simulink model "gm_DUALportRAMinterface_v3_vnl"  (R2024a)
settings: Solver=FixedStepDiscrete  StartTime=0.0  StopTime=20  RelTol=1e-3
undefined symbols (not defined in the file or in its folder): magnitude, Ts
libraries: hdlsllib x419, hdlmdlgenlib x103, embmathops x12, simulink x5, dsphdlxfrm2 x2
(part 2 of 11)

== system gm_DUALportRAMinterface_v3_vnl/PL/to_uint32_5 ==
  u_port : Inport  OutDataTypeStr=fixdt(1, 33, 15)  PortDimensions=1  SampleTime=3.00000003e-08
  Bit Concat : hdlsllib/Logic and Bit Operations/Bit Concat  numInputs=18
  Bit Shift1 : hdlsllib/Logic and Bit Operations/Bit Shift  mode=Shift Left Logical  N=15
  Bit Shift19 : hdlsllib/Logic and Bit Operations/Bit Shift  mode=Shift Left Logical  N=1
  Bit Shift2 : hdlsllib/Logic and Bit Operations/Bit Shift  mode=Shift Right Logical  N=16
  Bit Shift20 : hdlsllib/Logic and Bit Operations/Bit Shift  mode=Shift Left Logical  N=10
  Bit Shift21 : hdlsllib/Logic and Bit Operations/Bit Shift  mode=Shift Right Logical  N=1
  Bit Shift22 : hdlsllib/Logic and Bit Operations/Bit Shift  mode=Shift Left Logical  N=11
  Bit Shift23 : hdlsllib/Logic and Bit Operations/Bit Shift  mode=Shift Left Logical  N=12
  Bit Shift24 : hdlsllib/Logic and Bit Operations/Bit Shift  mode=Shift Left Logical  N=13
  Bit Shift25 : hdlsllib/Logic and Bit Operations/Bit Shift  mode=Shift Left Logical  N=14
  Bit Shift26 : hdlsllib/Logic and Bit Operations/Bit Shift  mode=Shift Left Logical  N=2
  Bit Shift27 : hdlsllib/Logic and Bit Operations/Bit Shift  mode=Shift Left Logical  N=3
  Bit Shift28 : hdlsllib/Logic and Bit Operations/Bit Shift  mode=Shift Left Logical  N=4
  Bit Shift29 : hdlsllib/Logic and Bit Operations/Bit Shift  mode=Shift Left Logical  N=5
  Bit Shift30 : hdlsllib/Logic and Bit Operations/Bit Shift  mode=Shift Left Logical  N=6
  Bit Shift31 : hdlsllib/Logic and Bit Operations/Bit Shift  mode=Shift Left Logical  N=7
  Bit Shift32 : hdlsllib/Logic and Bit Operations/Bit Shift  mode=Shift Left Logical  N=8
  Bit Shift33 : hdlsllib/Logic and Bit Operations/Bit Shift  mode=Shift Left Logical  N=9
  Data Type Conversion{1..2,12..16,26,34..43} (18 alike) : DataTypeConversion  OutDataTypeStr=fixdt(0,1,0)  SaturateOnIntegerOverflow=off  RndMeth=Floor
  Data Type Conversion44 : DataTypeConversion  OutDataTypeStr=uint32  SaturateOnIntegerOverflow=off  RndMeth=Floor
  Out1 : Outport  SampleTime=3.00000003e-08
  wires:
  Data Type Conversion44/1 -> Out1/1
  Data Type Conversion43/1 -> Bit Concat/10
  Data Type Conversion42/1 -> Bit Concat/12
  Data Type Conversion41/1 -> Bit Concat/13
  Data Type Conversion40/1 -> Bit Concat/14
  Data Type Conversion39/1 -> Bit Concat/15
  Data Type Conversion38/1 -> Bit Concat/16
  Data Type Conversion37/1 -> Bit Concat/17
  Data Type Conversion36/1 -> Bit Concat/4
  Data Type Conversion35/1 -> Bit Concat/5
  Data Type Conversion34/1 -> Bit Concat/6
  Data Type Conversion26/1 -> Bit Concat/7
  Data Type Conversion2/1 -> Bit Concat/1
  Data Type Conversion16/1 -> Bit Concat/8
  Data Type Conversion15/1 -> Bit Concat/9
  Data Type Conversion14/1 -> Bit Concat/11
  Data Type Conversion13/1 -> Bit Concat/2
  Data Type Conversion12/1 -> Bit Concat/3
  Data Type Conversion1/1 -> Bit Concat/18
  Bit Shift33/1 -> Data Type Conversion42/1
  Bit Shift32/1 -> Data Type Conversion14/1
  Bit Shift31/1 -> Data Type Conversion43/1
  Bit Shift30/1 -> Data Type Conversion15/1
  Bit Shift29/1 -> Data Type Conversion16/1
  Bit Shift28/1 -> Data Type Conversion26/1
  Bit Shift27/1 -> Data Type Conversion34/1
  Bit Shift26/1 -> Data Type Conversion35/1
  Bit Shift25/1 -> Data Type Conversion37/1
  Bit Shift24/1 -> Data Type Conversion38/1
  Bit Shift23/1 -> Data Type Conversion39/1
  Bit Shift22/1 -> Data Type Conversion40/1
  Bit Shift21/1 -> Data Type Conversion13/1
  Bit Shift20/1 -> Data Type Conversion41/1
  Bit Shift2/1 -> Data Type Conversion2/1
  Bit Shift19/1 -> Data Type Conversion36/1
  Bit Shift1/1 -> Data Type Conversion1/1
  Bit Concat/1 -> Data Type Conversion44/1
  u_port/1 -> Bit Shift1/1, Bit Shift19/1, Bit Shift2/1, Bit Shift20/1, Bit Shift21/1, Bit Shift22/1, Bit Shift23/1, Bit Shift24/1, Bit Shift25/1, Bit Shift26/1, Bit Shift27/1, Bit Shift28/1, Bit Shift29/1, Bit Shift30/1, Bit Shift31/1, Bit Shift32/1, Bit Shift33/1, Data Type Conversion12/1

== system gm_DUALportRAMinterface_v3_vnl/PL/to_uint32_6 ==
  u_port : Inport  OutDataTypeStr=fixdt(1, 33, 15)  PortDimensions=1  SampleTime=3.00000003e-08
  Bit Concat : hdlsllib/Logic and Bit Operations/Bit Concat  numInputs=18
  Bit Shift1 : hdlsllib/Logic and Bit Operations/Bit Shift  mode=Shift Left Logical  N=15
  Bit Shift19 : hdlsllib/Logic and Bit Operations/Bit Shift  mode=Shift Left Logical  N=1
  Bit Shift2 : hdlsllib/Logic and Bit Operations/Bit Shift  mode=Shift Right Logical  N=16
  Bit Shift20 : hdlsllib/Logic and Bit Operations/Bit Shift  mode=Shift Left Logical  N=10
  Bit Shift21 : hdlsllib/Logic and Bit Operations/Bit Shift  mode=Shift Right Logical  N=1
  Bit Shift22 : hdlsllib/Logic and Bit Operations/Bit Shift  mode=Shift Left Logical  N=11
  Bit Shift23 : hdlsllib/Logic and Bit Operations/Bit Shift  mode=Shift Left Logical  N=12
  Bit Shift24 : hdlsllib/Logic and Bit Operations/Bit Shift  mode=Shift Left Logical  N=13
  Bit Shift25 : hdlsllib/Logic and Bit Operations/Bit Shift  mode=Shift Left Logical  N=14
  Bit Shift26 : hdlsllib/Logic and Bit Operations/Bit Shift  mode=Shift Left Logical  N=2
  Bit Shift27 : hdlsllib/Logic and Bit Operations/Bit Shift  mode=Shift Left Logical  N=3
  Bit Shift28 : hdlsllib/Logic and Bit Operations/Bit Shift  mode=Shift Left Logical  N=4
  Bit Shift29 : hdlsllib/Logic and Bit Operations/Bit Shift  mode=Shift Left Logical  N=5
  Bit Shift30 : hdlsllib/Logic and Bit Operations/Bit Shift  mode=Shift Left Logical  N=6
  Bit Shift31 : hdlsllib/Logic and Bit Operations/Bit Shift  mode=Shift Left Logical  N=7
  Bit Shift32 : hdlsllib/Logic and Bit Operations/Bit Shift  mode=Shift Left Logical  N=8
  Bit Shift33 : hdlsllib/Logic and Bit Operations/Bit Shift  mode=Shift Left Logical  N=9
  Data Type Conversion{1..2,12..16,26,34..43} (18 alike) : DataTypeConversion  OutDataTypeStr=fixdt(0,1,0)  SaturateOnIntegerOverflow=off  RndMeth=Floor
  Data Type Conversion44 : DataTypeConversion  OutDataTypeStr=uint32  SaturateOnIntegerOverflow=off  RndMeth=Floor
  Out1 : Outport  SampleTime=3.00000003e-08
  wires:
  Data Type Conversion44/1 -> Out1/1
  Data Type Conversion43/1 -> Bit Concat/10
  Data Type Conversion42/1 -> Bit Concat/12
  Data Type Conversion41/1 -> Bit Concat/13
  Data Type Conversion40/1 -> Bit Concat/14
  Data Type Conversion39/1 -> Bit Concat/15
  Data Type Conversion38/1 -> Bit Concat/16
  Data Type Conversion37/1 -> Bit Concat/17
  Data Type Conversion36/1 -> Bit Concat/4
  Data Type Conversion35/1 -> Bit Concat/5
  Data Type Conversion34/1 -> Bit Concat/6
  Data Type Conversion26/1 -> Bit Concat/7
  Data Type Conversion2/1 -> Bit Concat/1
  Data Type Conversion16/1 -> Bit Concat/8
  Data Type Conversion15/1 -> Bit Concat/9
  Data Type Conversion14/1 -> Bit Concat/11
  Data Type Conversion13/1 -> Bit Concat/2
  Data Type Conversion12/1 -> Bit Concat/3
  Data Type Conversion1/1 -> Bit Concat/18
  Bit Shift33/1 -> Data Type Conversion42/1
  Bit Shift32/1 -> Data Type Conversion14/1
  Bit Shift31/1 -> Data Type Conversion43/1
  Bit Shift30/1 -> Data Type Conversion15/1
  Bit Shift29/1 -> Data Type Conversion16/1
  Bit Shift28/1 -> Data Type Conversion26/1
  Bit Shift27/1 -> Data Type Conversion34/1
  Bit Shift26/1 -> Data Type Conversion35/1
  Bit Shift25/1 -> Data Type Conversion37/1
  Bit Shift24/1 -> Data Type Conversion38/1
  Bit Shift23/1 -> Data Type Conversion39/1
  Bit Shift22/1 -> Data Type Conversion40/1
  Bit Shift21/1 -> Data Type Conversion13/1
  Bit Shift20/1 -> Data Type Conversion41/1
  Bit Shift2/1 -> Data Type Conversion2/1
  Bit Shift19/1 -> Data Type Conversion36/1
  Bit Shift1/1 -> Data Type Conversion1/1
  Bit Concat/1 -> Data Type Conversion44/1
  u_port/1 -> Bit Shift1/1, Bit Shift19/1, Bit Shift2/1, Bit Shift20/1, Bit Shift21/1, Bit Shift22/1, Bit Shift23/1, Bit Shift24/1, Bit Shift25/1, Bit Shift26/1, Bit Shift27/1, Bit Shift28/1, Bit Shift29/1, Bit Shift30/1, Bit Shift31/1, Bit Shift32/1, Bit Shift33/1, Data Type Conversion12/1

== system gm_DUALportRAMinterface_v3_vnl/PL_vnl/index_counter ==
  In1 : Inport
  In2 : Inport  Port=2
  Add : Sum  OutDataTypeStr=Inherit: Same as first input
  Constant18 : Constant  OutDataTypeStr=fixdt(0,16,0)  SampleTime=Ts
  Constant19 : Constant  Value=0  OutDataTypeStr=fixdt(0,16,0)  SampleTime=Ts
  Constant20 : Constant  Value=0  OutDataTypeStr=uint16  SampleTime=Ts
  Delay : Delay  DelayLength=1  InitialCondition=0  SampleTime=Ts
  Switch : Switch  Criteria=u2 > Threshold  SaturateOnIntegerOverflow=off  InputSameDT=off  OutDataTypeStr=Inherit: Same as first input
  Switch8 : Switch  Criteria=u2 > Threshold  SaturateOnIntegerOverflow=off  InputSameDT=off  OutDataTypeStr=Inherit: Same as first input
  index_counter : Outport
  wires:
  In1/1 -> Switch/2
  Constant18/1 -> Switch/1
  Constant20/1 -> Switch8/1
  Add/1 -> Delay/1
  In2/1 -> Switch8/2
  Delay/1 -> Switch8/3, index_counter/1
  Switch/1 -> Add/1
  Switch8/1 -> Add/2
  Constant19/1 -> Switch/3

== system gm_DUALportRAMinterface_v3_vnl/PL_vnl/integration_block1 ==
  data_in : Inport
  data_in1 : Inport  Port=2
  start_ga : Inport  Port=3
  D2 : Subsystem
      settings: PortSchema="{\"entries\":[{\"content\":{\"sides\":[{\"content\":{\"connectorIds\":[\"In1\",\"In2\"]},\"type\":\"ConnectorPlacement.EquallySpacedRectSide\",\"uuid\":\"5abe48ab-1b34-4cb0-8d41-07cb17904e64\"},{\"content\":{\"connectorIds\":[\"Out1\"],\"side\":\"RIGHT\"},\"type\":\"ConnectorPlacement.EquallySpacedRectSide\",\"uuid\":\"19bc24ff-88f3-42df-af8e-ecb9c1c6119c\"},{\"content\":{\"connectorIds\":[\"In3\"],\"side\":\"TOP\"},\"type\":\"ConnectorPlacement.EquallySpacedRectSide\",\"uuid\":\"46fc65c4-6cee-4e0a-9107-9d106d0a52a5\"},{\"content\":{\"connectorIds\":[\"In4\"],\"side\":\"BOTTOM\"},\"type\":\"ConnectorPlacement.EquallySpacedRectSide\",\"uuid\":\"10a5fc09-3948-4556-8b0c-050853396926\"}]},\"type\":\"ConnectorPlacement.EquallySpacedConnector\",\"uuid\":\"9cc35bfe-5b00-42b0-9811-425d4f0f8f7b\"}],\"packageUris\":[\"http://schema.mathworks.com/mf0/Connector/R2020b\"],\"version\":\"1.0\"}"
  Delay : Delay  DelayLength=6145  InitialCondition=0  UseCircularBuffer=on  SampleTime=Ts
  Delay3 : Delay  DelayLength=1  InitialCondition=0  SampleTime=Ts
  FFT : dsphdlxfrm2/FFT  Architecture=Burst Radix 2  FFTLengthSource=Property  FFTLength=4096  FFTLengthMax=1024  ComplexMultiplication=Use 4 multipliers and 2 adders  BitReversedOutput=off  BitReversedInput=off  Normalize=off  SimulateUsing=Code generation  RoundingMethod=Floor  ResetInputPort=on  StartOutputPort=off  EndOutputPort=off
  FIFO_system1 : Subsystem
  FIFO_system3 : Subsystem
  GA_main : Subsystem
      settings: PortSchema="{\"entries\":[{\"content\":{\"sides\":[{\"content\":{\"connectorIds\":[\"In1\",\"In2\",\"In3\",\"In4\",\"In5\",\"In6\",\"In7\",\"In8\",\"In9\",\"In10\",\"In11\"]},\"type\":\"ConnectorPlacement.EquallySpacedRectSide\",\"uuid\":\"daccc056-a93f-45e5-9369-71b73e32651e\"},{\"content\":{\"connectorIds\":[\"Out1\",\"Out2\"],\"side\":\"RIGHT\"},\"type\":\"ConnectorPlacement.EquallySpacedRectSide\",\"uuid\":\"82109161-9ebe-455f-914b-56f9927b10eb\"},{\"content\":{\"connectorIds\":[\"Out3\",\"Out4\",\"Out5\",\"In12\",\"In13\"],\"side\":\"TOP\"},\"type\":\"ConnectorPlacement.EquallySpacedRectSide\",\"uuid\":\"07b2e20b-bb92-4769-b746-3d44a115cdd8\"}]},\"type\":\"ConnectorPlacement.EquallySpacedConnector\",\"uuid\":\"c9f522d4-4f80-4900-b8a5-3110692e6ae8\"}],\"packageUris\":[\"http://schema.mathworks.com/mf0/Connector/R2020b\"],\"version\":\"1.0\"}"
  Scope1 : Scope
  Subsystem : Subsystem
  Sum : Sum  Inputs=|+-  OutDataTypeStr=Inherit: Same as first input
  Terminator : Terminator
  Terminator1 : Terminator
  Terminator2 : Terminator
  accumulator_scorer : Subsystem
  ga_done : Outport
  elite_individual : Outport  Port=2
  wires:
  GA_main/1(elite_individual) -> elite_individual/1
  FIFO_system1/4(FIFO_full) -> FIFO_system3/3(load_fifo)
  Subsystem/9(random_sample_out) -> GA_main/11(tb_random_sample)
  Subsystem/8(a4_random_out) -> GA_main/10(a4rnd)
  Subsystem/7(a3_random_out) -> GA_main/9(a3rnd)
  Subsystem/6(a2_random_out) -> GA_main/8(a2rnd)
  Subsystem/5(b4_random_out) -> GA_main/7(b4rnd)
  Subsystem/4(b3_random_out) -> GA_main/6(b3rnd)
  Subsystem/3(b2_random_out) -> GA_main/5(b2rnd)
  Subsystem/2(random_method_out) -> GA_main/4(random_method)
  Subsystem/1(random_gene_out) -> GA_main/3(random_gene)
  Delay/1 -> D2/3(reset_D2)
  Sum/1 -> FFT/1
  FIFO_system3/4(FIFO_full) -> GA_main/12(FIFO_full)
  FIFO_system1/3(reset_fft) -> FFT/3, Delay/1
  FIFO_system1/2(data_valid) -> FFT/2
  data_in1/1 -> FIFO_system3/1(data_in)
  Delay3/1 -> GA_main/13(score_done)
  FIFO_system3/3(reset_fft) -> Terminator2/1
  accumulator_scorer/2(individual_score_valid) -> Delay3/1
  GA_main/3(individual_to_d2) -> D2/4(Individual_input)
  FIFO_system3/1(data_out) -> D2/1(GAerror)
  GA_main/2(ga_done) -> ga_done/1
  data_in/1 -> FIFO_system1/1(data_in)
  GA_main/4(FIFO_out_en) -> FIFO_system1/2(enable_output), FIFO_system3/2(enable_output), D2/2(push_individual)
  GA_main/5(load_fifo) -> FIFO_system1/3(load_fifo)
  FFT/3 -> Terminator/1
  FFT/1 -> accumulator_scorer/1(data_in)
  D2/1(response) -> Sum/2
  start_ga/1 -> Subsystem/1(enable), GA_main/1(start_ga)
  FIFO_system1/1(data_out) -> Sum/1
  accumulator_scorer/1(individual_score) -> Scope1/1, GA_main/2(score_result)
  FIFO_system3/2(data_valid) -> Terminator1/1
  FFT/2 -> accumulator_scorer/2(valid_fft)

== system gm_DUALportRAMinterface_v3_vnl/PL_vnl/to_uint32_1 ==
  u_port : Inport
  Bit Concat : hdlsllib/Logic and Bit Operations/Bit Concat  numInputs=18
  Bit Shift1 : hdlsllib/Logic and Bit Operations/Bit Shift  mode=Shift Left Logical  N=15
  Bit Shift19 : hdlsllib/Logic and Bit Operations/Bit Shift  mode=Shift Left Logical  N=1
  Bit Shift2 : hdlsllib/Logic and Bit Operations/Bit Shift  mode=Shift Right Logical  N=16
  Bit Shift20 : hdlsllib/Logic and Bit Operations/Bit Shift  mode=Shift Left Logical  N=10
  Bit Shift21 : hdlsllib/Logic and Bit Operations/Bit Shift  mode=Shift Right Logical  N=1
  Bit Shift22 : hdlsllib/Logic and Bit Operations/Bit Shift  mode=Shift Left Logical  N=11
  Bit Shift23 : hdlsllib/Logic and Bit Operations/Bit Shift  mode=Shift Left Logical  N=12
  Bit Shift24 : hdlsllib/Logic and Bit Operations/Bit Shift  mode=Shift Left Logical  N=13
  Bit Shift25 : hdlsllib/Logic and Bit Operations/Bit Shift  mode=Shift Left Logical  N=14
  Bit Shift26 : hdlsllib/Logic and Bit Operations/Bit Shift  mode=Shift Left Logical  N=2
  Bit Shift27 : hdlsllib/Logic and Bit Operations/Bit Shift  mode=Shift Left Logical  N=3
  Bit Shift28 : hdlsllib/Logic and Bit Operations/Bit Shift  mode=Shift Left Logical  N=4
  Bit Shift29 : hdlsllib/Logic and Bit Operations/Bit Shift  mode=Shift Left Logical  N=5
  Bit Shift30 : hdlsllib/Logic and Bit Operations/Bit Shift  mode=Shift Left Logical  N=6
  Bit Shift31 : hdlsllib/Logic and Bit Operations/Bit Shift  mode=Shift Left Logical  N=7
  Bit Shift32 : hdlsllib/Logic and Bit Operations/Bit Shift  mode=Shift Left Logical  N=8
  Bit Shift33 : hdlsllib/Logic and Bit Operations/Bit Shift  mode=Shift Left Logical  N=9
  Data Type Conversion{1..2,12..16,26,34..43} (18 alike) : DataTypeConversion  OutDataTypeStr=fixdt(0,1,0)  SaturateOnIntegerOverflow=off  RndMeth=Floor
  Data Type Conversion44 : DataTypeConversion  OutDataTypeStr=uint32  SaturateOnIntegerOverflow=off  RndMeth=Floor
  Out1 : Outport
  wires:
  Bit Concat/1 -> Data Type Conversion44/1
  u_port/1 -> Bit Shift1/1, Bit Shift21/1, Bit Shift2/1, Data Type Conversion12/1, Bit Shift19/1, Bit Shift26/1, Bit Shift27/1, Bit Shift28/1, Bit Shift29/1, Bit Shift30/1, Bit Shift31/1, Bit Shift32/1, Bit Shift33/1, Bit Shift20/1, Bit Shift22/1, Bit Shift23/1, Bit Shift24/1, Bit Shift25/1
  Data Type Conversion14/1 -> Bit Concat/11
  Data Type Conversion1/1 -> Bit Concat/18
  Data Type Conversion2/1 -> Bit Concat/1
  Data Type Conversion26/1 -> Bit Concat/7
  Bit Shift21/1 -> Data Type Conversion13/1
  Data Type Conversion12/1 -> Bit Concat/3
  Bit Shift27/1 -> Data Type Conversion34/1
  Bit Shift22/1 -> Data Type Conversion40/1
  Bit Shift20/1 -> Data Type Conversion41/1
  Bit Shift31/1 -> Data Type Conversion43/1
  Data Type Conversion39/1 -> Bit Concat/15
  Data Type Conversion15/1 -> Bit Concat/9
  Data Type Conversion43/1 -> Bit Concat/10
  Bit Shift33/1 -> Data Type Conversion42/1
  Bit Shift23/1 -> Data Type Conversion39/1
  Bit Shift25/1 -> Data Type Conversion37/1
  Data Type Conversion41/1 -> Bit Concat/13
  Bit Shift2/1 -> Data Type Conversion2/1
  Bit Shift29/1 -> Data Type Conversion16/1
  Bit Shift26/1 -> Data Type Conversion35/1
  Data Type Conversion34/1 -> Bit Concat/6
  Bit Shift28/1 -> Data Type Conversion26/1
  Data Type Conversion36/1 -> Bit Concat/4
  Bit Shift24/1 -> Data Type Conversion38/1
  Bit Shift1/1 -> Data Type Conversion1/1
  Data Type Conversion35/1 -> Bit Concat/5
  Data Type Conversion16/1 -> Bit Concat/8
  Bit Shift19/1 -> Data Type Conversion36/1
  Data Type Conversion13/1 -> Bit Concat/2
  Bit Shift30/1 -> Data Type Conversion15/1
  Data Type Conversion38/1 -> Bit Concat/16
  Data Type Conversion37/1 -> Bit Concat/17
  Data Type Conversion40/1 -> Bit Concat/14
  Bit Shift32/1 -> Data Type Conversion14/1
  Data Type Conversion42/1 -> Bit Concat/12
  Data Type Conversion44/1 -> Out1/1

== system gm_DUALportRAMinterface_v3_vnl/PL_vnl/to_uint32_2 ==
  u_port : Inport
  Bit Concat : hdlsllib/Logic and Bit Operations/Bit Concat  numInputs=18
  Bit Shift1 : hdlsllib/Logic and Bit Operations/Bit Shift  mode=Shift Left Logical  N=15
  Bit Shift19 : hdlsllib/Logic and Bit Operations/Bit Shift  mode=Shift Left Logical  N=1
  Bit Shift2 : hdlsllib/Logic and Bit Operations/Bit Shift  mode=Shift Right Logical  N=16
  Bit Shift20 : hdlsllib/Logic and Bit Operations/Bit Shift  mode=Shift Left Logical  N=10
  Bit Shift21 : hdlsllib/Logic and Bit Operations/Bit Shift  mode=Shift Right Logical  N=1
  Bit Shift22 : hdlsllib/Logic and Bit Operations/Bit Shift  mode=Shift Left Logical  N=11
  Bit Shift23 : hdlsllib/Logic and Bit Operations/Bit Shift  mode=Shift Left Logical  N=12
  Bit Shift24 : hdlsllib/Logic and Bit Operations/Bit Shift  mode=Shift Left Logical  N=13
  Bit Shift25 : hdlsllib/Logic and Bit Operations/Bit Shift  mode=Shift Left Logical  N=14
  Bit Shift26 : hdlsllib/Logic and Bit Operations/Bit Shift  mode=Shift Left Logical  N=2
  Bit Shift27 : hdlsllib/Logic and Bit Operations/Bit Shift  mode=Shift Left Logical  N=3
  Bit Shift28 : hdlsllib/Logic and Bit Operations/Bit Shift  mode=Shift Left Logical  N=4
  Bit Shift29 : hdlsllib/Logic and Bit Operations/Bit Shift  mode=Shift Left Logical  N=5
  Bit Shift30 : hdlsllib/Logic and Bit Operations/Bit Shift  mode=Shift Left Logical  N=6
  Bit Shift31 : hdlsllib/Logic and Bit Operations/Bit Shift  mode=Shift Left Logical  N=7
  Bit Shift32 : hdlsllib/Logic and Bit Operations/Bit Shift  mode=Shift Left Logical  N=8
  Bit Shift33 : hdlsllib/Logic and Bit Operations/Bit Shift  mode=Shift Left Logical  N=9
  Data Type Conversion{1..2,12..16,26,34..43} (18 alike) : DataTypeConversion  OutDataTypeStr=fixdt(0,1,0)  SaturateOnIntegerOverflow=off  RndMeth=Floor
  Data Type Conversion44 : DataTypeConversion  OutDataTypeStr=uint32  SaturateOnIntegerOverflow=off  RndMeth=Floor
  Out1 : Outport
  wires:
  Data Type Conversion44/1 -> Out1/1
  Data Type Conversion42/1 -> Bit Concat/12
  Bit Shift32/1 -> Data Type Conversion14/1
  Data Type Conversion40/1 -> Bit Concat/14
  Data Type Conversion37/1 -> Bit Concat/17
  Data Type Conversion38/1 -> Bit Concat/16
  Bit Shift30/1 -> Data Type Conversion15/1
  Data Type Conversion13/1 -> Bit Concat/2
  Bit Shift19/1 -> Data Type Conversion36/1
  Data Type Conversion16/1 -> Bit Concat/8
  Data Type Conversion35/1 -> Bit Concat/5
  Bit Shift1/1 -> Data Type Conversion1/1
  Bit Shift24/1 -> Data Type Conversion38/1
  Data Type Conversion36/1 -> Bit Concat/4
  Bit Shift28/1 -> Data Type Conversion26/1
  Data Type Conversion34/1 -> Bit Concat/6
  Bit Shift26/1 -> Data Type Conversion35/1
  Bit Shift29/1 -> Data Type Conversion16/1
  Bit Shift2/1 -> Data Type Conversion2/1
  Data Type Conversion41/1 -> Bit Concat/13
  Bit Shift25/1 -> Data Type Conversion37/1
  Bit Shift23/1 -> Data Type Conversion39/1
  Bit Shift33/1 -> Data Type Conversion42/1
  Data Type Conversion43/1 -> Bit Concat/10
  Data Type Conversion15/1 -> Bit Concat/9
  Data Type Conversion39/1 -> Bit Concat/15
  Bit Shift31/1 -> Data Type Conversion43/1
  Bit Shift20/1 -> Data Type Conversion41/1
  Bit Shift22/1 -> Data Type Conversion40/1
  Bit Shift27/1 -> Data Type Conversion34/1
  Data Type Conversion12/1 -> Bit Concat/3
  Bit Shift21/1 -> Data Type Conversion13/1
  Data Type Conversion26/1 -> Bit Concat/7
  Data Type Conversion2/1 -> Bit Concat/1
  Data Type Conversion1/1 -> Bit Concat/18
  Data Type Conversion14/1 -> Bit Concat/11
  u_port/1 -> Bit Shift25/1, Bit Shift24/1, Bit Shift23/1, Bit Shift22/1, Bit Shift20/1, Bit Shift33/1, Bit Shift32/1, Bit Shift31/1, Bit Shift30/1, Bit Shift29/1, Bit Shift28/1, Bit Shift27/1, Bit Shift26/1, Bit Shift19/1, Data Type Conversion12/1, Bit Shift2/1, Bit Shift21/1, Bit Shift1/1
  Bit Concat/1 -> Data Type Conversion44/1

== system gm_DUALportRAMinterface_v3_vnl/PL_vnl/to_uint32_3 ==
  u_port : Inport
  Bit Concat : hdlsllib/Logic and Bit Operations/Bit Concat  numInputs=18
  Bit Shift1 : hdlsllib/Logic and Bit Operations/Bit Shift  mode=Shift Left Logical  N=15
  Bit Shift19 : hdlsllib/Logic and Bit Operations/Bit Shift  mode=Shift Left Logical  N=1
  Bit Shift2 : hdlsllib/Logic and Bit Operations/Bit Shift  mode=Shift Right Logical  N=16
  Bit Shift20 : hdlsllib/Logic and Bit Operations/Bit Shift  mode=Shift Left Logical  N=10
  Bit Shift21 : hdlsllib/Logic and Bit Operations/Bit Shift  mode=Shift Right Logical  N=1
  Bit Shift22 : hdlsllib/Logic and Bit Operations/Bit Shift  mode=Shift Left Logical  N=11
  Bit Shift23 : hdlsllib/Logic and Bit Operations/Bit Shift  mode=Shift Left Logical  N=12
  Bit Shift24 : hdlsllib/Logic and Bit Operations/Bit Shift  mode=Shift Left Logical  N=13
  Bit Shift25 : hdlsllib/Logic and Bit Operations/Bit Shift  mode=Shift Left Logical  N=14
  Bit Shift26 : hdlsllib/Logic and Bit Operations/Bit Shift  mode=Shift Left Logical  N=2
  Bit Shift27 : hdlsllib/Logic and Bit Operations/Bit Shift  mode=Shift Left Logical  N=3
  Bit Shift28 : hdlsllib/Logic and Bit Operations/Bit Shift  mode=Shift Left Logical  N=4
  Bit Shift29 : hdlsllib/Logic and Bit Operations/Bit Shift  mode=Shift Left Logical  N=5
  Bit Shift30 : hdlsllib/Logic and Bit Operations/Bit Shift  mode=Shift Left Logical  N=6
  Bit Shift31 : hdlsllib/Logic and Bit Operations/Bit Shift  mode=Shift Left Logical  N=7
  Bit Shift32 : hdlsllib/Logic and Bit Operations/Bit Shift  mode=Shift Left Logical  N=8
  Bit Shift33 : hdlsllib/Logic and Bit Operations/Bit Shift  mode=Shift Left Logical  N=9
  Data Type Conversion{1..2,12..16,26,34..43} (18 alike) : DataTypeConversion  OutDataTypeStr=fixdt(0,1,0)  SaturateOnIntegerOverflow=off  RndMeth=Floor
  Data Type Conversion44 : DataTypeConversion  OutDataTypeStr=uint32  SaturateOnIntegerOverflow=off  RndMeth=Floor
  Out1 : Outport
  wires:
  Bit Concat/1 -> Data Type Conversion44/1
  u_port/1 -> Bit Shift1/1, Bit Shift21/1, Bit Shift2/1, Data Type Conversion12/1, Bit Shift19/1, Bit Shift26/1, Bit Shift27/1, Bit Shift28/1, Bit Shift29/1, Bit Shift30/1, Bit Shift31/1, Bit Shift32/1, Bit Shift33/1, Bit Shift20/1, Bit Shift22/1, Bit Shift23/1, Bit Shift24/1, Bit Shift25/1
  Data Type Conversion14/1 -> Bit Concat/11
  Data Type Conversion1/1 -> Bit Concat/18
  Data Type Conversion2/1 -> Bit Concat/1
  Data Type Conversion26/1 -> Bit Concat/7
  Bit Shift21/1 -> Data Type Conversion13/1
  Data Type Conversion12/1 -> Bit Concat/3
  Bit Shift27/1 -> Data Type Conversion34/1
  Bit Shift22/1 -> Data Type Conversion40/1
  Bit Shift20/1 -> Data Type Conversion41/1
  Bit Shift31/1 -> Data Type Conversion43/1
  Data Type Conversion39/1 -> Bit Concat/15
  Data Type Conversion15/1 -> Bit Concat/9
  Data Type Conversion43/1 -> Bit Concat/10
  Bit Shift33/1 -> Data Type Conversion42/1
  Bit Shift23/1 -> Data Type Conversion39/1
  Bit Shift25/1 -> Data Type Conversion37/1
  Data Type Conversion41/1 -> Bit Concat/13
  Bit Shift2/1 -> Data Type Conversion2/1
  Bit Shift29/1 -> Data Type Conversion16/1
  Bit Shift26/1 -> Data Type Conversion35/1
  Data Type Conversion34/1 -> Bit Concat/6
  Bit Shift28/1 -> Data Type Conversion26/1
  Data Type Conversion36/1 -> Bit Concat/4
  Bit Shift24/1 -> Data Type Conversion38/1
  Bit Shift1/1 -> Data Type Conversion1/1
  Data Type Conversion35/1 -> Bit Concat/5
  Data Type Conversion16/1 -> Bit Concat/8
  Bit Shift19/1 -> Data Type Conversion36/1
  Data Type Conversion13/1 -> Bit Concat/2
  Bit Shift30/1 -> Data Type Conversion15/1
  Data Type Conversion38/1 -> Bit Concat/16
  Data Type Conversion37/1 -> Bit Concat/17
  Data Type Conversion40/1 -> Bit Concat/14
  Bit Shift32/1 -> Data Type Conversion14/1
  Data Type Conversion42/1 -> Bit Concat/12
  Data Type Conversion44/1 -> Out1/1

== system gm_DUALportRAMinterface_v3_vnl/PL_vnl/to_uint32_4 ==
  u_port : Inport
  Bit Concat : hdlsllib/Logic and Bit Operations/Bit Concat  numInputs=18
  Bit Shift1 : hdlsllib/Logic and Bit Operations/Bit Shift  mode=Shift Left Logical  N=15
  Bit Shift19 : hdlsllib/Logic and Bit Operations/Bit Shift  mode=Shift Left Logical  N=1
  Bit Shift2 : hdlsllib/Logic and Bit Operations/Bit Shift  mode=Shift Right Logical  N=16
  Bit Shift20 : hdlsllib/Logic and Bit Operations/Bit Shift  mode=Shift Left Logical  N=10
  Bit Shift21 : hdlsllib/Logic and Bit Operations/Bit Shift  mode=Shift Right Logical  N=1
  Bit Shift22 : hdlsllib/Logic and Bit Operations/Bit Shift  mode=Shift Left Logical  N=11
  Bit Shift23 : hdlsllib/Logic and Bit Operations/Bit Shift  mode=Shift Left Logical  N=12
  Bit Shift24 : hdlsllib/Logic and Bit Operations/Bit Shift  mode=Shift Left Logical  N=13
  Bit Shift25 : hdlsllib/Logic and Bit Operations/Bit Shift  mode=Shift Left Logical  N=14
  Bit Shift26 : hdlsllib/Logic and Bit Operations/Bit Shift  mode=Shift Left Logical  N=2
  Bit Shift27 : hdlsllib/Logic and Bit Operations/Bit Shift  mode=Shift Left Logical  N=3
  Bit Shift28 : hdlsllib/Logic and Bit Operations/Bit Shift  mode=Shift Left Logical  N=4
  Bit Shift29 : hdlsllib/Logic and Bit Operations/Bit Shift  mode=Shift Left Logical  N=5
  Bit Shift30 : hdlsllib/Logic and Bit Operations/Bit Shift  mode=Shift Left Logical  N=6
  Bit Shift31 : hdlsllib/Logic and Bit Operations/Bit Shift  mode=Shift Left Logical  N=7
  Bit Shift32 : hdlsllib/Logic and Bit Operations/Bit Shift  mode=Shift Left Logical  N=8
  Bit Shift33 : hdlsllib/Logic and Bit Operations/Bit Shift  mode=Shift Left Logical  N=9
  Data Type Conversion{1..2,12..16,26,34..43} (18 alike) : DataTypeConversion  OutDataTypeStr=fixdt(0,1,0)  SaturateOnIntegerOverflow=off  RndMeth=Floor
  Data Type Conversion44 : DataTypeConversion  OutDataTypeStr=uint32  SaturateOnIntegerOverflow=off  RndMeth=Floor
  Out1 : Outport
  wires:
  Data Type Conversion44/1 -> Out1/1
  Data Type Conversion42/1 -> Bit Concat/12
  Bit Shift32/1 -> Data Type Conversion14/1
  Data Type Conversion40/1 -> Bit Concat/14
  Data Type Conversion37/1 -> Bit Concat/17
  Data Type Conversion38/1 -> Bit Concat/16
  Bit Shift30/1 -> Data Type Conversion15/1
  Data Type Conversion13/1 -> Bit Concat/2
  Bit Shift19/1 -> Data Type Conversion36/1
  Data Type Conversion16/1 -> Bit Concat/8
  Data Type Conversion35/1 -> Bit Concat/5
  Bit Shift1/1 -> Data Type Conversion1/1
  Bit Shift24/1 -> Data Type Conversion38/1
  Data Type Conversion36/1 -> Bit Concat/4
  Bit Shift28/1 -> Data Type Conversion26/1
  Data Type Conversion34/1 -> Bit Concat/6
  Bit Shift26/1 -> Data Type Conversion35/1
  Bit Shift29/1 -> Data Type Conversion16/1
  Bit Shift2/1 -> Data Type Conversion2/1
  Data Type Conversion41/1 -> Bit Concat/13
  Bit Shift25/1 -> Data Type Conversion37/1
  Bit Shift23/1 -> Data Type Conversion39/1
  Bit Shift33/1 -> Data Type Conversion42/1
  Data Type Conversion43/1 -> Bit Concat/10
  Data Type Conversion15/1 -> Bit Concat/9
  Data Type Conversion39/1 -> Bit Concat/15
  Bit Shift31/1 -> Data Type Conversion43/1
  Bit Shift20/1 -> Data Type Conversion41/1
  Bit Shift22/1 -> Data Type Conversion40/1
  Bit Shift27/1 -> Data Type Conversion34/1
  Data Type Conversion12/1 -> Bit Concat/3
  Bit Shift21/1 -> Data Type Conversion13/1
  Data Type Conversion26/1 -> Bit Concat/7
  Data Type Conversion2/1 -> Bit Concat/1
  Data Type Conversion1/1 -> Bit Concat/18
  Data Type Conversion14/1 -> Bit Concat/11
  u_port/1 -> Bit Shift25/1, Bit Shift24/1, Bit Shift23/1, Bit Shift22/1, Bit Shift20/1, Bit Shift33/1, Bit Shift32/1, Bit Shift31/1, Bit Shift30/1, Bit Shift29/1, Bit Shift28/1, Bit Shift27/1, Bit Shift26/1, Bit Shift19/1, Data Type Conversion12/1, Bit Shift2/1, Bit Shift21/1, Bit Shift1/1
  Bit Concat/1 -> Data Type Conversion44/1

== system gm_DUALportRAMinterface_v3_vnl/PL_vnl/to_uint32_5 ==
  u_port : Inport
  Bit Concat : hdlsllib/Logic and Bit Operations/Bit Concat  numInputs=18
  Bit Shift1 : hdlsllib/Logic and Bit Operations/Bit Shift  mode=Shift Left Logical  N=15
  Bit Shift19 : hdlsllib/Logic and Bit Operations/Bit Shift  mode=Shift Left Logical  N=1
  Bit Shift2 : hdlsllib/Logic and Bit Operations/Bit Shift  mode=Shift Right Logical  N=16
  Bit Shift20 : hdlsllib/Logic and Bit Operations/Bit Shift  mode=Shift Left Logical  N=10
  Bit Shift21 : hdlsllib/Logic and Bit Operations/Bit Shift  mode=Shift Right Logical  N=1
  Bit Shift22 : hdlsllib/Logic and Bit Operations/Bit Shift  mode=Shift Left Logical  N=11
  Bit Shift23 : hdlsllib/Logic and Bit Operations/Bit Shift  mode=Shift Left Logical  N=12
  Bit Shift24 : hdlsllib/Logic and Bit Operations/Bit Shift  mode=Shift Left Logical  N=13
  Bit Shift25 : hdlsllib/Logic and Bit Operations/Bit Shift  mode=Shift Left Logical  N=14
  Bit Shift26 : hdlsllib/Logic and Bit Operations/Bit Shift  mode=Shift Left Logical  N=2
  Bit Shift27 : hdlsllib/Logic and Bit Operations/Bit Shift  mode=Shift Left Logical  N=3
  Bit Shift28 : hdlsllib/Logic and Bit Operations/Bit Shift  mode=Shift Left Logical  N=4
  Bit Shift29 : hdlsllib/Logic and Bit Operations/Bit Shift  mode=Shift Left Logical  N=5
  Bit Shift30 : hdlsllib/Logic and Bit Operations/Bit Shift  mode=Shift Left Logical  N=6
  Bit Shift31 : hdlsllib/Logic and Bit Operations/Bit Shift  mode=Shift Left Logical  N=7
  Bit Shift32 : hdlsllib/Logic and Bit Operations/Bit Shift  mode=Shift Left Logical  N=8
  Bit Shift33 : hdlsllib/Logic and Bit Operations/Bit Shift  mode=Shift Left Logical  N=9
  Data Type Conversion{1..2,12..16,26,34..43} (18 alike) : DataTypeConversion  OutDataTypeStr=fixdt(0,1,0)  SaturateOnIntegerOverflow=off  RndMeth=Floor
  Data Type Conversion44 : DataTypeConversion  OutDataTypeStr=uint32  SaturateOnIntegerOverflow=off  RndMeth=Floor
  Out1 : Outport
  wires:
  Bit Concat/1 -> Data Type Conversion44/1
  u_port/1 -> Bit Shift1/1, Bit Shift21/1, Bit Shift2/1, Data Type Conversion12/1, Bit Shift19/1, Bit Shift26/1, Bit Shift27/1, Bit Shift28/1, Bit Shift29/1, Bit Shift30/1, Bit Shift31/1, Bit Shift32/1, Bit Shift33/1, Bit Shift20/1, Bit Shift22/1, Bit Shift23/1, Bit Shift24/1, Bit Shift25/1
  Data Type Conversion14/1 -> Bit Concat/11
  Data Type Conversion1/1 -> Bit Concat/18
  Data Type Conversion2/1 -> Bit Concat/1
  Data Type Conversion26/1 -> Bit Concat/7
  Bit Shift21/1 -> Data Type Conversion13/1
  Data Type Conversion12/1 -> Bit Concat/3
  Bit Shift27/1 -> Data Type Conversion34/1
  Bit Shift22/1 -> Data Type Conversion40/1
  Bit Shift20/1 -> Data Type Conversion41/1
  Bit Shift31/1 -> Data Type Conversion43/1
  Data Type Conversion39/1 -> Bit Concat/15
  Data Type Conversion15/1 -> Bit Concat/9
  Data Type Conversion43/1 -> Bit Concat/10
  Bit Shift33/1 -> Data Type Conversion42/1
  Bit Shift23/1 -> Data Type Conversion39/1
  Bit Shift25/1 -> Data Type Conversion37/1
  Data Type Conversion41/1 -> Bit Concat/13
  Bit Shift2/1 -> Data Type Conversion2/1
  Bit Shift29/1 -> Data Type Conversion16/1
  Bit Shift26/1 -> Data Type Conversion35/1
  Data Type Conversion34/1 -> Bit Concat/6
  Bit Shift28/1 -> Data Type Conversion26/1
  Data Type Conversion36/1 -> Bit Concat/4
  Bit Shift24/1 -> Data Type Conversion38/1
  Bit Shift1/1 -> Data Type Conversion1/1
  Data Type Conversion35/1 -> Bit Concat/5
  Data Type Conversion16/1 -> Bit Concat/8
  Bit Shift19/1 -> Data Type Conversion36/1
  Data Type Conversion13/1 -> Bit Concat/2
  Bit Shift30/1 -> Data Type Conversion15/1
  Data Type Conversion38/1 -> Bit Concat/16
  Data Type Conversion37/1 -> Bit Concat/17
  Data Type Conversion40/1 -> Bit Concat/14
  Bit Shift32/1 -> Data Type Conversion14/1
  Data Type Conversion42/1 -> Bit Concat/12
  Data Type Conversion44/1 -> Out1/1

== system gm_DUALportRAMinterface_v3_vnl/PL_vnl/to_uint32_6 ==
  u_port : Inport
  Bit Concat : hdlsllib/Logic and Bit Operations/Bit Concat  numInputs=18
  Bit Shift1 : hdlsllib/Logic and Bit Operations/Bit Shift  mode=Shift Left Logical  N=15
  Bit Shift19 : hdlsllib/Logic and Bit Operations/Bit Shift  mode=Shift Left Logical  N=1
  Bit Shift2 : hdlsllib/Logic and Bit Operations/Bit Shift  mode=Shift Right Logical  N=16
  Bit Shift20 : hdlsllib/Logic and Bit Operations/Bit Shift  mode=Shift Left Logical  N=10
  Bit Shift21 : hdlsllib/Logic and Bit Operations/Bit Shift  mode=Shift Right Logical  N=1
  Bit Shift22 : hdlsllib/Logic and Bit Operations/Bit Shift  mode=Shift Left Logical  N=11
  Bit Shift23 : hdlsllib/Logic and Bit Operations/Bit Shift  mode=Shift Left Logical  N=12
  Bit Shift24 : hdlsllib/Logic and Bit Operations/Bit Shift  mode=Shift Left Logical  N=13
  Bit Shift25 : hdlsllib/Logic and Bit Operations/Bit Shift  mode=Shift Left Logical  N=14
  Bit Shift26 : hdlsllib/Logic and Bit Operations/Bit Shift  mode=Shift Left Logical  N=2
  Bit Shift27 : hdlsllib/Logic and Bit Operations/Bit Shift  mode=Shift Left Logical  N=3
  Bit Shift28 : hdlsllib/Logic and Bit Operations/Bit Shift  mode=Shift Left Logical  N=4
  Bit Shift29 : hdlsllib/Logic and Bit Operations/Bit Shift  mode=Shift Left Logical  N=5
  Bit Shift30 : hdlsllib/Logic and Bit Operations/Bit Shift  mode=Shift Left Logical  N=6
  Bit Shift31 : hdlsllib/Logic and Bit Operations/Bit Shift  mode=Shift Left Logical  N=7
  Bit Shift32 : hdlsllib/Logic and Bit Operations/Bit Shift  mode=Shift Left Logical  N=8
  Bit Shift33 : hdlsllib/Logic and Bit Operations/Bit Shift  mode=Shift Left Logical  N=9
  Data Type Conversion{1..2,12..16,26,34..43} (18 alike) : DataTypeConversion  OutDataTypeStr=fixdt(0,1,0)  SaturateOnIntegerOverflow=off  RndMeth=Floor
  Data Type Conversion44 : DataTypeConversion  OutDataTypeStr=uint32  SaturateOnIntegerOverflow=off  RndMeth=Floor
  Out1 : Outport
  wires:
  Data Type Conversion44/1 -> Out1/1
  Data Type Conversion42/1 -> Bit Concat/12
  Bit Shift32/1 -> Data Type Conversion14/1
  Data Type Conversion40/1 -> Bit Concat/14
  Data Type Conversion37/1 -> Bit Concat/17
  Data Type Conversion38/1 -> Bit Concat/16
  Bit Shift30/1 -> Data Type Conversion15/1
  Data Type Conversion13/1 -> Bit Concat/2
  Bit Shift19/1 -> Data Type Conversion36/1
  Data Type Conversion16/1 -> Bit Concat/8
  Data Type Conversion35/1 -> Bit Concat/5
  Bit Shift1/1 -> Data Type Conversion1/1
  Bit Shift24/1 -> Data Type Conversion38/1
  Data Type Conversion36/1 -> Bit Concat/4
  Bit Shift28/1 -> Data Type Conversion26/1
  Data Type Conversion34/1 -> Bit Concat/6
  Bit Shift26/1 -> Data Type Conversion35/1
  Bit Shift29/1 -> Data Type Conversion16/1
  Bit Shift2/1 -> Data Type Conversion2/1
  Data Type Conversion41/1 -> Bit Concat/13
  Bit Shift25/1 -> Data Type Conversion37/1
  Bit Shift23/1 -> Data Type Conversion39/1
  Bit Shift33/1 -> Data Type Conversion42/1
  Data Type Conversion43/1 -> Bit Concat/10
  Data Type Conversion15/1 -> Bit Concat/9
  Data Type Conversion39/1 -> Bit Concat/15
  Bit Shift31/1 -> Data Type Conversion43/1
  Bit Shift20/1 -> Data Type Conversion41/1
  Bit Shift22/1 -> Data Type Conversion40/1
  Bit Shift27/1 -> Data Type Conversion34/1
  Data Type Conversion12/1 -> Bit Concat/3
  Bit Shift21/1 -> Data Type Conversion13/1
  Data Type Conversion26/1 -> Bit Concat/7
  Data Type Conversion2/1 -> Bit Concat/1
  Data Type Conversion1/1 -> Bit Concat/18
  Data Type Conversion14/1 -> Bit Concat/11
  u_port/1 -> Bit Shift25/1, Bit Shift24/1, Bit Shift23/1, Bit Shift22/1, Bit Shift20/1, Bit Shift33/1, Bit Shift32/1, Bit Shift31/1, Bit Shift30/1, Bit Shift29/1, Bit Shift28/1, Bit Shift27/1, Bit Shift26/1, Bit Shift19/1, Data Type Conversion12/1, Bit Shift2/1, Bit Shift21/1, Bit Shift1/1
  Bit Concat/1 -> Data Type Conversion44/1

== system gm_DUALportRAMinterface_v3_vnl/PL/integration_block1/D2 ==
  GAerror : Inport  OutDataTypeStr=fixdt(1, 16, 14)  PortDimensions=1  SampleTime=3.00000003e-08
  push_individual : Inport  Port=2  OutDataTypeStr=boolean  PortDimensions=1  SampleTime=3.00000003e-08
  reset_D2 : Inport  Port=3  OutDataTypeStr=boolean  PortDimensions=1  SampleTime=3.00000003e-08
  Individual_input : Inport  Port=4  OutDataTypeStr=fixdt(1, 33, 15)  PortDimensions=[7]  SampleTime=3.00000003e-08
  Product{,1..5} (6 alike) : Product  Inputs=**  OutDataTypeStr=fixdt(1, 64, 32)  SampleTime=3.00000003e-08
  denom_acc11 : Sum  Inputs=+-  OutDataTypeStr=fixdt(1, 64, 32)  AccumDataTypeStr=fixdt(1, 64, 32)  SampleTime=3.00000003e-08
  denom_acc2 : Sum  Inputs=+-  OutDataTypeStr=fixdt(1, 64, 32)  AccumDataTypeStr=fixdt(1, 64, 32)  SampleTime=3.00000003e-08
  denom_acc3 : Sum  Inputs=+-  OutDataTypeStr=fixdt(1, 64, 32)  AccumDataTypeStr=fixdt(1, 64, 32)  SampleTime=3.00000003e-08
  individual1 : Subsystem
  individual1_term0 : Terminator
  output_cast1 : Subsystem  mask(Buffer/Wire){}
      mask help: Buffer
  reset_sw{,1..6} (7 alike) : Switch  Criteria=u2 > Threshold  Threshold=double(0)  OutDataTypeStr=fixdt(1, 64, 32)  SampleTime=3.00000003e-08  SaturateOnIntegerOverflow=off  InputSameDT=off
  s_nume_acc11 : Sum  OutDataTypeStr=fixdt(1, 64, 32)  AccumDataTypeStr=fixdt(1, 65, 32)  SampleTime=3.00000003e-08
  s_nume_acc2 : Sum  OutDataTypeStr=fixdt(1, 64, 32)  AccumDataTypeStr=fixdt(1, 65, 32)  SampleTime=3.00000003e-08
  s_nume_acc3 : Sum  OutDataTypeStr=fixdt(1, 14, 12)  AccumDataTypeStr=fixdt(1, 65, 32)  SampleTime=3.00000003e-08
  s_state_out11 : Delay  DelayLength=double(1)  InitialCondition=0  SampleTime=3.00000003e-08
  s_state_out2 : Delay  DelayLength=double(1)  InitialCondition=0  SampleTime=3.00000003e-08
  s_state_out3 : Delay  DelayLength=double(1)  InitialCondition=0  SampleTime=3.00000003e-08
  t : Demux  Outputs=7
  zero{,1..6} (7 alike) : Constant  Value="fi(0,1,64,32,\"hex\",\"0000000000000000\")"  OutDataTypeStr=fixdt(1, 64, 32)  SampleTime=3.00000003e-08
  response : Outport  SampleTime=3.00000003e-08
  wires:
  denom_acc2/1 -> denom_acc3/1
  denom_acc11/1 -> denom_acc2/1
  reset_sw6/1 -> denom_acc11/2
  Product2/1 -> reset_sw6/3
  reset_sw5/1 -> denom_acc2/2
  Product1/1 -> reset_sw5/3
  reset_sw4/1 -> denom_acc3/2
  Product/1 -> reset_sw4/3
  GAerror/1 -> denom_acc11/1
  zero4/1 -> reset_sw6/1
  individual1/5(b2) -> Product2/2
  zero5/1 -> reset_sw5/1
  individual1/6(b3) -> Product1/2
  zero6/1 -> reset_sw4/1
  individual1/7(b4) -> Product/2
  t/7 -> individual1/7(reg_in6)
  t/6 -> individual1/6(reg_in5)
  t/5 -> individual1/5(reg_in4)
  t/4 -> individual1/4(reg_in3)
  t/3 -> individual1/3(reg_in2)
  t/2 -> individual1/2(reg_in1)
  t/1 -> individual1/1(reg_in)
  individual1/1(score) -> individual1_term0/1
  zero3/1 -> reset_sw3/1
  zero2/1 -> reset_sw2/1
  zero1/1 -> reset_sw1/1
  zero/1 -> reset_sw/1
  s_state_out3/1 -> Product/1, Product3/1
  s_state_out2/1 -> Product1/1, s_state_out3/1, Product4/1
  s_state_out11/1 -> Product2/1, s_state_out2/1, Product5/1
  s_nume_acc3/1 -> output_cast1/1(in)
  s_nume_acc2/1 -> s_nume_acc3/1
  s_nume_acc11/1 -> s_nume_acc2/1
  reset_sw3/1 -> s_nume_acc11/1
  reset_sw2/1 -> s_nume_acc3/2
  reset_sw1/1 -> s_nume_acc2/2
  reset_sw/1 -> s_nume_acc11/2
  output_cast1/1(out) -> response/1
  individual1/4(a4) -> Product3/2
  individual1/3(a3) -> Product4/2
  individual1/2(a2) -> Product5/2
  denom_acc3/1 -> s_state_out11/1, reset_sw3/3
  Product5/1 -> reset_sw/3
  Product4/1 -> reset_sw1/3
  Product3/1 -> reset_sw2/3
  Individual_input/1 -> t/1
  reset_D2/1 -> reset_sw4/2, reset_sw5/2, reset_sw6/2, reset_sw/2, reset_sw1/2, reset_sw2/2, reset_sw3/2
  push_individual/1 -> individual1/8(enable)

== system gm_DUALportRAMinterface_v3_vnl/PL/integration_block1/FIFO_system1 ==
  data_in : Inport  OutDataTypeStr=fixdt(1, 16, 14)  PortDimensions=1  SampleTime=3.00000003e-08
  enable_output : Inport  Port=2  OutDataTypeStr=boolean  PortDimensions=1  SampleTime=3.00000003e-08
  load_fifo : Inport  Port=3  OutDataTypeStr=boolean  PortDimensions=1  SampleTime=3.00000003e-08
  Add1 : Sum  OutDataTypeStr=fixdt(0,13,0)
  Chart1 : Subsystem
  Chart2 : Subsystem
  Chart3 : Subsystem
  Constant3 : Constant  OutDataTypeStr=fixdt(0,12,0)  SampleTime=Ts
  Constant4 : Constant  Value=0  OutDataTypeStr=fixdt(1,13,0)  SampleTime=Ts
  Delay : Delay  DelayLength=2048  InitialCondition=0  UseCircularBuffer=on
  Delay1 : Delay  DelayLength=1  InitialCondition=0  SampleTime=Ts
  Delay2 : Delay  DelayLength=1  InitialCondition=0  SampleTime=Ts
  Delay3 : Delay  DelayLength=1  InitialCondition=0
  HDL FIFO1 : hdlsllib/HDL RAMs/HDL FIFO  fifo_size=4096+2048+1  mode=Classic  ratio=1  push_msg=Warning  pop_msg=Warning  show_empty=off  show_full=on  show_num=off  LabelModeActiveChoice_Mode=Classic  rst_port=off
  Logical Operator : Logic  Operator=OR  IconShape=distinctive  AllPortsSameDT=off  OutDataTypeStr=boolean
  Logical Operator1 : Logic  IconShape=distinctive  AllPortsSameDT=off  OutDataTypeStr=boolean
  Logical Operator2 : Logic  IconShape=distinctive  AllPortsSameDT=off  OutDataTypeStr=boolean
  Logical Operator3 : Logic  Operator=XOR  IconShape=distinctive  AllPortsSameDT=off  OutDataTypeStr=boolean
  Logical Operator4 : Logic  IconShape=distinctive  AllPortsSameDT=off  OutDataTypeStr=boolean
  Logical Operator5 : Logic  Operator=XOR  IconShape=distinctive  AllPortsSameDT=off  OutDataTypeStr=boolean
  Logical Operator6 : Logic  Operator=XOR  IconShape=distinctive  AllPortsSameDT=off  OutDataTypeStr=boolean
  Switch1 : Switch  Criteria=u2 ~= 0  OutDataTypeStr=fixdt(0,13,0)  SaturateOnIntegerOverflow=off  InputSameDT=off
  Switch3 : Switch  Criteria=u2 ~= 0  OutDataTypeStr=fixdt(1, 16, 14)  SaturateOnIntegerOverflow=off  InputSameDT=off
  tuneback : Delay  DelayLength=2048+4096+0  InitialCondition=0  UseCircularBuffer=on
  data_out : Outport  SampleTime=3.00000003e-08
  data_valid : Outport  Port=2  SampleTime=3.00000003e-08
  reset_fft : Outport  Port=3  SampleTime=3.00000003e-08
  FIFO_full : Outport  Port=4  SampleTime=3.00000003e-08
  wires:
  Add1/1 -> Switch1/1
  Chart1/1(enable_counter) -> Switch1/2
  Constant3/1 -> Add1/2
  Constant4/1 -> Switch1/3
  enable_output/1 -> Chart1/2(en_out)
  Delay1/1 -> Add1/1, Chart1/1(counter)
  Switch3/1 -> HDL FIFO1/1
  Chart2/1(enable_push) -> Logical Operator/1, Switch3/2
  Logical Operator/1 -> HDL FIFO1/2
  tuneback/1 -> Logical Operator4/2
  Switch1/1 -> Delay1/1, Chart3/1(counter)
  Logical Operator6/1 -> FIFO_full/1
  Logical Operator5/1 -> data_valid/1
  Logical Operator4/1 -> Logical Operator5/2
  Logical Operator3/1 -> reset_fft/1
  Logical Operator2/1 -> Logical Operator3/1, Logical Operator5/1
  Logical Operator1/1 -> Delay/1, tuneback/1, Logical Operator2/1, Logical Operator3/2, Logical Operator4/1
  HDL FIFO1/2 -> Chart2/2(full), Delay3/1, Logical Operator6/1
  HDL FIFO1/1 -> Switch3/3, data_out/1
  Delay3/1 -> Logical Operator6/2
  Delay2/1 -> Logical Operator1/2
  Delay/1 -> Logical Operator2/2
  Chart3/1(enable_pop) -> HDL FIFO1/3, Logical Operator/2, Delay2/1, Logical Operator1/1
  load_fifo/1 -> Chart2/1(load_FIFO1)
  data_in/1 -> Switch3/1

== system gm_DUALportRAMinterface_v3_vnl/PL/integration_block1/FIFO_system3 ==
  data_in : Inport  OutDataTypeStr=fixdt(1, 16, 14)  PortDimensions=1  SampleTime=3.00000003e-08
  enable_output : Inport  Port=2  OutDataTypeStr=boolean  PortDimensions=1  SampleTime=3.00000003e-08
  load_fifo : Inport  Port=3  OutDataTypeStr=boolean  PortDimensions=1  SampleTime=3.00000003e-08
  Add1 : Sum  OutDataTypeStr=fixdt(0,13,0)
  Chart1 : Subsystem
  Chart2 : Subsystem
  Chart3 : Subsystem
  Constant3 : Constant  OutDataTypeStr=fixdt(0,12,0)  SampleTime=Ts
  Constant4 : Constant  Value=0  OutDataTypeStr=fixdt(1,13,0)  SampleTime=Ts
  Delay1 : Delay  DelayLength=1  InitialCondition=0  SampleTime=Ts
  Delay3 : Delay  DelayLength=1  InitialCondition=0
  HDL FIFO1 : hdlsllib/HDL RAMs/HDL FIFO  fifo_size=4096+2048+1  mode=Classic  ratio=1  push_msg=Warning  pop_msg=Warning  show_empty=off  show_full=on  show_num=off  LabelModeActiveChoice_Mode=Classic  rst_port=off
  Logical Operator : Logic  Operator=OR  IconShape=distinctive  AllPortsSameDT=off  OutDataTypeStr=boolean
  Logical Operator6 : Logic  Operator=XOR  IconShape=distinctive  AllPortsSameDT=off  OutDataTypeStr=boolean
  Switch1 : Switch  Criteria=u2 ~= 0  OutDataTypeStr=fixdt(0,13,0)  SaturateOnIntegerOverflow=off  InputSameDT=off
  Switch3 : Switch  Criteria=u2 ~= 0  OutDataTypeStr=fixdt(1, 16, 14)  SaturateOnIntegerOverflow=off  InputSameDT=off
  t : Constant  Value=double(0)  OutDataTypeStr=boolean  SampleTime=3.00000003e-08
  t1 : Constant  Value=double(0)  OutDataTypeStr=boolean  SampleTime=3.00000003e-08
  data_out : Outport  SampleTime=3.00000003e-08
  data_valid : Outport  Port=2  SampleTime=3.00000003e-08
  reset_fft : Outport  Port=3  SampleTime=3.00000003e-08
  FIFO_full : Outport  Port=4  SampleTime=3.00000003e-08
  wires:
  Add1/1 -> Switch1/1
  Chart1/1(enable_counter) -> Switch1/2
  Constant3/1 -> Add1/2
  Constant4/1 -> Switch1/3
  enable_output/1 -> Chart1/2(en_out)
  Delay1/1 -> Add1/1, Chart1/1(counter)
  Switch3/1 -> HDL FIFO1/1
  Chart2/1(enable_push) -> Logical Operator/1, Switch3/2
  Logical Operator/1 -> HDL FIFO1/2
  Switch1/1 -> Delay1/1, Chart3/1(counter)
  Logical Operator6/1 -> FIFO_full/1
  t/1 -> data_valid/1
  t1/1 -> reset_fft/1
  HDL FIFO1/2 -> Chart2/2(full), Delay3/1, Logical Operator6/1
  HDL FIFO1/1 -> Switch3/3, data_out/1
  Delay3/1 -> Logical Operator6/2
  Chart3/1(enable_pop) -> HDL FIFO1/3, Logical Operator/2
  load_fifo/1 -> Chart2/1(load_FIFO1)
  data_in/1 -> Switch3/1
